simulink model "H7_1GDL_Lineal_filtro"  (R2022b)
settings: Solver=VariableStepAuto  StartTime=0.0  StopTime=10  RelTol=1e-3
model workspace (MAT data in the model file):
  surfaceBlockParameters = Simulink.LookupTable
  surfaceBlockParameters.Table = Simulink.lookuptable.Table
  surfaceBlockParameters.Table.Value = [145.669360614  122.326612109  101.996418654  84.6787802495  70.3736968941  59.0811685884  50.8011953324  45.5337771261  43.2789139695  44.0366058625; 185.313749978  156.270189263  130.473313595  107.923122972  88.6196173961  72.5627968658  59.7526613816  50.1892109434  43.8724455513  40.8023652052; 237.482290208  203.298417321  172.595359476  145.373116673  121.631688913  101.371076195  84.59127852  71.2922958872  61.4741282968  55.1367757489; 296.780859506  258.017174483  222.968434498  191.634639553  164.015789646  140.111884779  119.92292495  103.44891016  90.6898404082  81.6457156957; 357.815336073  315.032338952  276.198416866  241.313569815  210.377797799  183.391100818  160.353478873  141.264931963  126.125460088  114.935063248; 415.191598113  368.94978893  326.891184779  289.01578566  255.323591572  225.814602516  200.488818491  179.346239498  162.386865537  149.610696607; 463.515523826  414.37540262  369.652616441  329.347165291  293.459049169  261.988268074  234.934822007  212.298710969  194.079934958  180.278493975; 497.392991416  445.915058223  399.088590054  356.91358691  319.39004879  286.517975694  258.297367623  234.728224576  215.810546553  201.544333555; 511.429879083  458.174633941  409.804983819  366.320928719  327.722468638  294.009603579  265.18233354  241.240658522  222.184578525  208.014093548]
  surfaceBlockParameters.Table.Dimensions = [9 10]
  surfaceBlockParameters.Table.DataType = 'auto'
  surfaceBlockParameters.Table.FieldName = 'Table_force'
  surfaceBlockParameters.Breakpoints(1) = Simulink.lookuptable.Breakpoint
  surfaceBlockParameters.Breakpoints(1).Value = [-40 -31.1 -22.2 -13.3 -4.4 4.5 13.4 22.3 31.2]
  surfaceBlockParameters.Breakpoints(1).TunableSizeName = 'N1'
  surfaceBlockParameters.Breakpoints(1).Dimensions = [1 9]
  surfaceBlockParameters.Breakpoints(1).DataType = 'auto'
  surfaceBlockParameters.Breakpoints(1).FieldName = 'BP1_current'
  surfaceBlockParameters.Breakpoints(2) = Simulink.lookuptable.Breakpoint
  surfaceBlockParameters.Breakpoints(2).Value = [0.011 0.0123 0.0136 0.0149 0.0162 0.0175 0.0188 0.0201 0.0214 0.0227]
  surfaceBlockParameters.Breakpoints(2).TunableSizeName = 'N2'
  surfaceBlockParameters.Breakpoints(2).Dimensions = [1 10]
  surfaceBlockParameters.Breakpoints(2).DataType = 'auto'
  surfaceBlockParameters.Breakpoints(2).FieldName = 'BP2_airgap'
  surfaceBlockParameters.AllowMultipleInstancesOfTypeToHaveDifferentTableBreakpointSizes = 0
  surfaceBlockParameters.SupportTunableSize = 0
  surfaceBlockParameters.StructTypeInfo = Simulink.lookuptable.StructTypeInfo
  surfaceBlockParameters.StructTypeInfo.Name = 'surfaceBlockParameters_type'
  surfaceBlockParameters.StructTypeInfo.DataScope = 'Auto'
values from neighbouring files (symbols this model uses):
  A = argout.a    [h7_nolineal.m]
  B = argout.b    [h7_nolineal.m]
  C = argout.c    [h7_nolineal.m]
  D = argout.d    [h7_nolineal.m]
libraries: slpidlib x2, simulink x1, cstblocks x1, dspstat3 x1
settings Model: Creator=USUARIO  LastModifiedBy=aceao

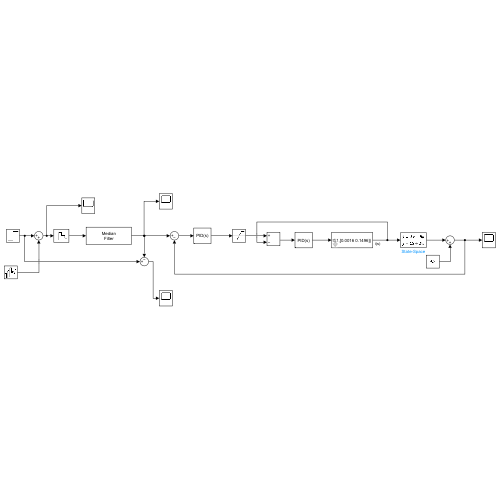
[thumbnail: Simulink's stored preview of the top-level diagram]
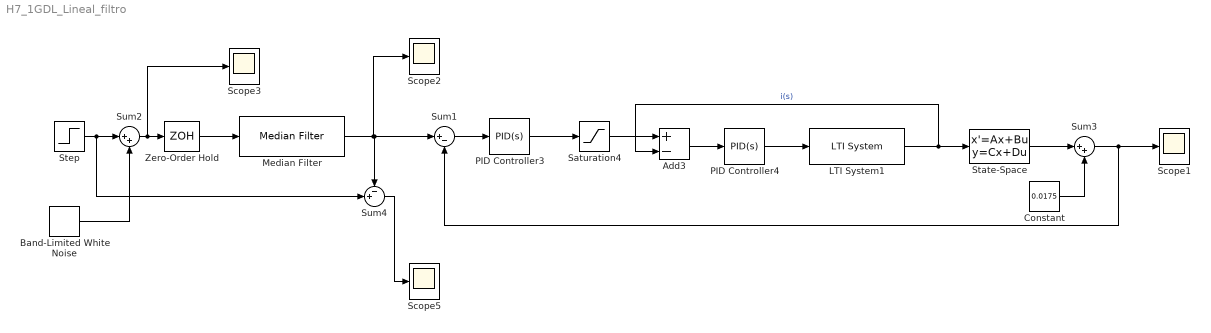
== system H7_1GDL_Lineal_filtro ==
  Add3 : Sum  Inputs=+-
  Band-Limited White Noise : simulink/Sources/Band-Limited White Noise  Cov=[0.0000000001]  Ts=0.001  seed=[2]
  Constant : Constant  Value=0.0175
  LTI System1 : cstblocks/LTI System  sys=tf(1,[0.0016 0.1496])  IC=[]
  Median Filter : dspstat3/Median Filter  WindowLength=10  SimulateUsing=Interpreted execution
      settings: LibrarySourceBlock=|
      | dspfdesign/Median
      | Filter
  PID Controller3 : slpidlib/PID Controller  Controller=PID  Form=Parallel  TimeDomain=Continuous-time  UseExternalTs=off  SampleTime=-1  IntegratorMethod=Forward Euler  FilterMethod=Forward Euler  ControllerParametersSource=internal  P=-90039.5075843937  I=-1426732.21591299  UseKiTs=off  D=-1395.2982301274  N=1846.03168412766  UseFilter=on  TunerSelectOption=Transfer Function Based (PID Tuner App)  InitialConditionSource=internal  InitialConditionForIntegrator=0  InitialConditionForFilter=0  DifferentiatorICPrevScaledInput=0  ExternalReset=none  TrackingMode=off  Kt=1  LimitOutput=off  SatLimitsSource=internal  UpperSaturationLimit=inf  LowerSaturationLimit=-inf  LinearizeAsGain=on  AntiWindupMode=none  Kb=1  LimitIntegrator=off  UpperIntegratorSaturationLimit=inf  LowerIntegratorSaturationLimit=-inf  POutMin=[]  POutMax=[]  IOutMin=[]  IOutMax=[]  DOutMin=[]  DOutMax=[]  NOutMin=[]  NOutMax=[]  SumOutMin=[]  SumOutMax=[]  SaturationOutMin=[]  SaturationOutMax=[]  PParamMin=[]  PParamMax=[]  IParamMin=[]  IParamMax=[]  DParamMin=[]  DParamMax=[]  NParamMin=[]  NParamMax=[]  KbParamMin=[]  KbParamMax=[]  KtParamMin=[]  KtParamMax=[]  KbOutMin=[]  KbOutMax=[]  KtOutMin=[]  KtOutMax=[]  IntegratorOutMin=[]  IntegratorOutMax=[]  FilterOutMin=[]  FilterOutMax=[]  SumI1OutMin=[]  SumI1OutMax=[]  SumI2OutMin=[]  SumI2OutMax=[]  SumI3OutMin=[]  SumI3OutMax=[]  SumI4OutMin=[]  SumI4OutMax=[]  SumDOutMin=[]  SumDOutMax=[]  DifferentiatorOutMin=[]  DifferentiatorOutMax=[]  FilterDiffOutCoefMin=[]  FilterDiffOutCoefMax=[]  ReciprocalOutMin=[]  ReciprocalOutMax=[]  SumDenOutMin=[]  SumDenOutMax=[]  SumNumOutMin=[]  SumNumOutMax=[]  DivideOutMin=[]  DivideOutMax=[]  UdiffTsProdOutMin=[]  UdiffTsProdOutMax=[]  NTsProdOutMin=[]  NTsProdOutMax=[]  UintegralTsProdOutMin=[]  UintegralTsProdOutMax=[]  UngainTsProdOutMin=[]  UngainTsProdOutMax=[]  ClampingZeroOutDataTypeStr=Inherit: Inherit via back propagation  ClampingZeroOutMin=[]  ClampingZeroOutMax=[]  FilterDenConstantOutDataTypeStr=Inherit: Inherit via back propagation  FilterDenConstantOutMin=[]  FilterDenConstantOutMax=[]  PCopyOutDataTypeStr=Inherit: Inherit via back propagation  PCopyOutMin=[]  PCopyOutMax=[]  NCopyOutDataTypeStr=Inherit: Inherit via back propagation  NCopyOutMin=[]  NCopyOutMax=[]  IntegratorContinuousStateAttributes=''  IntegratorStateMustResolveToSignalObject=off  IntegratorRTWStateStorageClass=Auto  FilterContinuousStateAttributes=''  FilterStateMustResolveToSignalObject=off  FilterRTWStateStorageClass=Auto  ParallelPVariant=InternalParameters  IdealPVariant=Disabled  IVariant=InternalParameters  DVariant=InternalParameters  IntegratorVariant=Continuous  SatVariant=Disabled  AWVariant=Passthrough  PCopyVariant=Disabled  TRVariant=Disabled  FdbkBlocksVariant=Forward  IdealPFdbkVariant=Disabled  SatFdbkVariant=Disabled  DerivativeFilterVariant=ContFilter  NVariant=InternalParameters  NCopyVariant=Disabled  FilterICVariant=InternalICsFilter  IntegratorICVariant=InternalICs  ExternalResetVariant=Disabled  TRSumVariant=Passthrough  SumFdbkVariant=Disabled  SumVariant=Sum_PID  TsampFilterVariant=InternalTs  TsampNgainVariant=Passthrough  TsampIntegralVariant=Passthrough  ExternalSaturationOutDataTypeStr=Inherit: Same as second input
  PID Controller4 : slpidlib/PID Controller  Controller=PID  Form=Parallel  TimeDomain=Continuous-time  UseExternalTs=off  SampleTime=-1  IntegratorMethod=Forward Euler  FilterMethod=Forward Euler  ControllerParametersSource=internal  P=2.9609617421093  I=472.321773987356  UseKiTs=off  D=-1.54969230406852e-05  N=191067.719336005  UseFilter=on  TunerSelectOption=Transfer Function Based (PID Tuner App)  InitialConditionSource=internal  InitialConditionForIntegrator=0  InitialConditionForFilter=0  DifferentiatorICPrevScaledInput=0  ExternalReset=none  TrackingMode=off  Kt=1  LimitOutput=off  SatLimitsSource=internal  UpperSaturationLimit=inf  LowerSaturationLimit=-inf  LinearizeAsGain=on  AntiWindupMode=none  Kb=1  LimitIntegrator=off  UpperIntegratorSaturationLimit=inf  LowerIntegratorSaturationLimit=-inf  POutMin=[]  POutMax=[]  IOutMin=[]  IOutMax=[]  DOutMin=[]  DOutMax=[]  NOutMin=[]  NOutMax=[]  SumOutMin=[]  SumOutMax=[]  SaturationOutMin=[]  SaturationOutMax=[]  PParamMin=[]  PParamMax=[]  IParamMin=[]  IParamMax=[]  DParamMin=[]  DParamMax=[]  NParamMin=[]  NParamMax=[]  KbParamMin=[]  KbParamMax=[]  KtParamMin=[]  KtParamMax=[]  KbOutMin=[]  KbOutMax=[]  KtOutMin=[]  KtOutMax=[]  IntegratorOutMin=[]  IntegratorOutMax=[]  FilterOutMin=[]  FilterOutMax=[]  SumI1OutMin=[]  SumI1OutMax=[]  SumI2OutMin=[]  SumI2OutMax=[]  SumI3OutMin=[]  SumI3OutMax=[]  SumI4OutMin=[]  SumI4OutMax=[]  SumDOutMin=[]  SumDOutMax=[]  DifferentiatorOutMin=[]  DifferentiatorOutMax=[]  FilterDiffOutCoefMin=[]  FilterDiffOutCoefMax=[]  ReciprocalOutMin=[]  ReciprocalOutMax=[]  SumDenOutMin=[]  SumDenOutMax=[]  SumNumOutMin=[]  SumNumOutMax=[]  DivideOutMin=[]  DivideOutMax=[]  UdiffTsProdOutMin=[]  UdiffTsProdOutMax=[]  NTsProdOutMin=[]  NTsProdOutMax=[]  UintegralTsProdOutMin=[]  UintegralTsProdOutMax=[]  UngainTsProdOutMin=[]  UngainTsProdOutMax=[]  ClampingZeroOutDataTypeStr=Inherit: Inherit via back propagation  ClampingZeroOutMin=[]  ClampingZeroOutMax=[]  FilterDenConstantOutDataTypeStr=Inherit: Inherit via back propagation  FilterDenConstantOutMin=[]  FilterDenConstantOutMax=[]  PCopyOutDataTypeStr=Inherit: Inherit via back propagation  PCopyOutMin=[]  PCopyOutMax=[]  NCopyOutDataTypeStr=Inherit: Inherit via back propagation  NCopyOutMin=[]  NCopyOutMax=[]  IntegratorContinuousStateAttributes=''  IntegratorStateMustResolveToSignalObject=off  IntegratorRTWStateStorageClass=Auto  FilterContinuousStateAttributes=''  FilterStateMustResolveToSignalObject=off  FilterRTWStateStorageClass=Auto  ParallelPVariant=InternalParameters  IdealPVariant=Disabled  IVariant=InternalParameters  DVariant=InternalParameters  IntegratorVariant=Continuous  SatVariant=Disabled  AWVariant=Passthrough  PCopyVariant=Disabled  TRVariant=Disabled  FdbkBlocksVariant=Forward  IdealPFdbkVariant=Disabled  SatFdbkVariant=Disabled  DerivativeFilterVariant=ContFilter  NVariant=InternalParameters  NCopyVariant=Disabled  FilterICVariant=InternalICsFilter  IntegratorICVariant=InternalICs  ExternalResetVariant=Disabled  TRSumVariant=Passthrough  SumFdbkVariant=Disabled  SumVariant=Sum_PID  TsampFilterVariant=InternalTs  TsampNgainVariant=Passthrough  TsampIntegralVariant=Passthrough  ExternalSaturationOutDataTypeStr=Inherit: Same as second input
  Saturation4 : Saturate  UpperLimit=40  LowerLimit=-40
  Scope{1..3,5} (4 alike) : Scope
  State-Space : StateSpace  A=A  B=B  C=C  D=D  InitialCondition=0
  Step : Step  Before=0.0175  After=0.0185  SampleTime=0
  Sum1 : Sum  Inputs=|+-
  Sum2 : Sum  Inputs=|++
  Sum3 : Sum  Inputs=|++
  Sum4 : Sum  Inputs=-+|
  Zero-Order Hold : ZeroOrderHold  SampleTime=0.01
  wires:
  Sum1/1 -> PID Controller3/1
  Saturation4/1 -> Add3/1
  LTI System1/1 -> State-Space/1, Add3/2  "i(s)"
  PID Controller4/1 -> LTI System1/1
  Add3/1 -> PID Controller4/1
  PID Controller3/1 -> Saturation4/1
  State-Space/1 -> Sum3/1
  Sum3/1 -> Scope1/1, Sum1/2
  Constant/1 -> Sum3/2
  Step/1 -> Sum4/2, Sum2/1
  Sum2/1 -> Zero-Order Hold/1, Scope3/1
  Band-Limited White Noise/1 -> Sum2/2
  Zero-Order Hold/1 -> Median Filter/1
  Median Filter/1 -> Sum4/1, Sum1/1, Scope2/1
  Sum4/1 -> Scope5/1
